simulink model "loopshape_id"  (Simulink 9.3)
settings: Solver=ode45  StartTime=0.0  StopTime=10.0  RelTol=1e-3  EnableMultiTasking=on
values from neighbouring files (symbols this model uses):
  Cs = 0.3    [Copy_of_mainCT.m]    (also in mainCT.m; testct.m = 0.1)
settings Model: Creator=felipe  LastModifiedBy=lakat
settings DataIOCC: LimitDataPoints=on  SignalLoggingSaveFormat=Dataset
settings DebuggingCC: UnderspecifiedInitializationDetection=Simplified  MergeDetectMultiDrivingBlocksExec=error  SolverPrmCheckMsg=warning  FcnCallInpInsideContextMsg=error
settings HardwareCC: TargetBitPerPointer=64  TargetBitPerSizeT=64  TargetBitPerPtrDiffT=64  TargetLongLongMode=on  TargetIntDivRoundTo=Zero  TargetEndianess=LittleEndian  TargetWordSize=64  TargetHWDeviceType=MATLAB Host  ProdEqTarget=off
settings RTWCC: SystemTargetFile=rtwsfcn.tlc  TemplateMakefile=rtwsfcn_default_tmf  Description=S-Function Target  TargetLang=C++
settings STFCustomTargetCC: ModelReferenceCompliant=off  CompOptLevelCompliant=on  MATLABClassNameForMDSCustomization=Simulink.SoftwareTarget.TargetSpecificTriggerConfigurationBase  SystemTargetFile=rtwsfcn.tlc
settings CustomProperty: Value=on

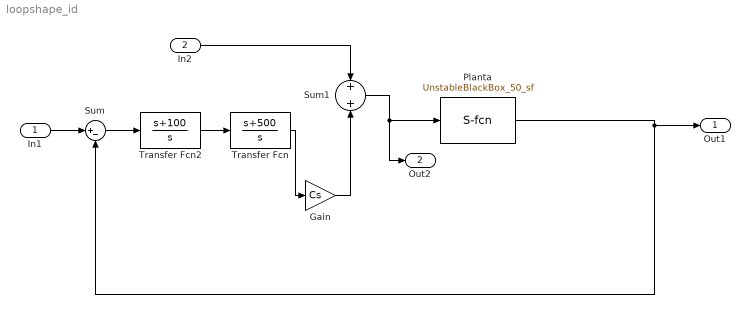
== system loopshape_id ==
  In1 : Inport
  In2 : Inport  Port=2
  Gain : Gain  Gain=Cs
  Planta : S-Function  FunctionName=UnstableBlackBox_50_sf  SFunctionDeploymentMode=off  EnableBusSupport=off  SFcnStateName=DWORK0
      settings: SFcnIsStateOwnerBlock=on
  Sum : Sum  Inputs=|+-
  Sum1 : Sum
  Transfer Fcn : TransferFcn  Numerator=[1 500]  Denominator=[1 0]
  Transfer Fcn2 : TransferFcn  Numerator=[1 100]  Denominator=[1 0]
  Out1 : Outport
  Out2 : Outport  Port=2
  wires:
  In1/1 -> Sum/1
  In2/1 -> Sum1/1
  Gain/1 -> Sum1/2
  Sum1/1 -> Out2/1, Planta/1
  Planta/1 -> Out1/1, Sum/2
  Transfer Fcn2/1 -> Transfer Fcn/1
  Sum/1 -> Transfer Fcn2/1
  Transfer Fcn/1 -> Gain/1
